simulink model "adm"  (R2020a)
settings: Solver=FixedStepAuto  StartTime=0.0  StopTime=2  FixedStep=0.00005  RelTol=1e-3
libraries: simulink x14, fuzblock x3
settings Model: Creator=13228  LastModifiedBy=13228
settings SolverCC: ZeroCrossAlgorithm=Adaptive

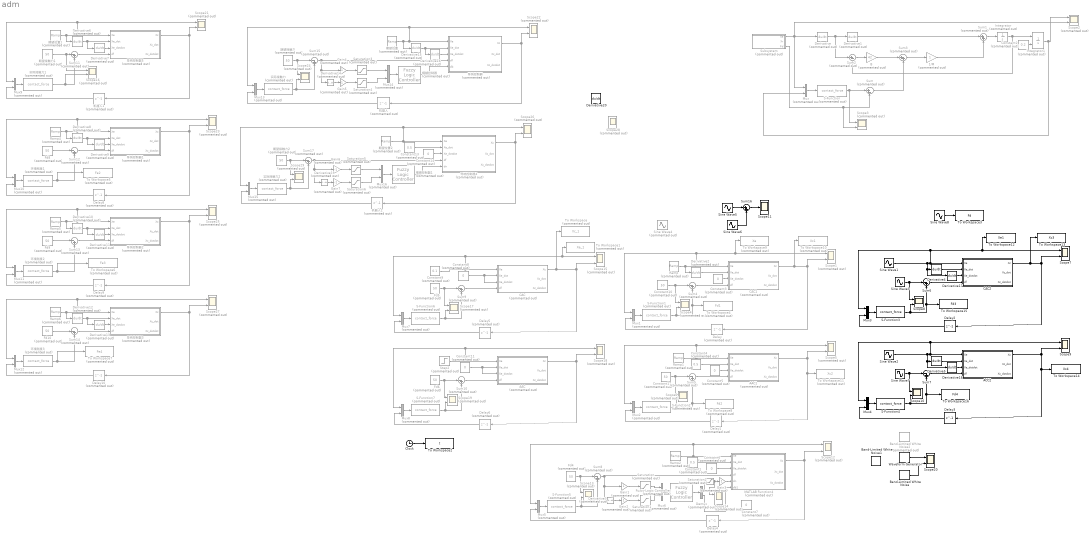
== system adm ==
  1/M : Gain  Commented=on
  AAC : MATLAB Function  Commented=on  TreatAsAtomicUnit=on
  AAC1 : MATLAB Function  Commented=on  TreatAsAtomicUnit=on
  ACC2 : MATLAB Function  TreatAsAtomicUnit=on
  B : Gain  Commented=on  Gain=42
  Band-Limited White Noise : simulink/Sources/Band-Limited White Noise  Cov=[0.2*0.2*0.01]  Ts=0.01  seed=[23341]
  Band-Limited White Noise1 : simulink/Sources/Band-Limited White Noise  Cov=[0.1]  Ts=0.1  seed=[23341]
  Band-Limited White Noise2 : simulink/Sources/Band-Limited White Noise  Commented=on  Cov=[0.1]  Ts=0.1  seed=[23341]
  CAC : MATLAB Function  Commented=on  TreatAsAtomicUnit=on
  CAC1 : MATLAB Function  Commented=on  TreatAsAtomicUnit=on
  CAC2 : MATLAB Function  TreatAsAtomicUnit=on
  Clock : Clock
  Constant1 : Constant  Commented=on  Value=0.5
  Constant10 : Constant  Commented=on  Value=50
  Constant{3,5..8,11,14} (7 alike) : Constant  Commented=on  Value=0
  Constant12 : Constant  Commented=on  Value=50
  Constant13 : Constant  Commented=on  Value=0.5
  Constant2 : Constant  Commented=on  Value=0.2
  Constant4 : Constant  Commented=on  Value=0.5
  Constant9 : Constant  Commented=on  Value=0.1
  Delay{,1,4,8..10} (6 alike) : Delay  Commented=on  DelayLength=1  InitialCondition=-0.002
  Delay2 : Delay  DelayLength=1  InitialCondition=0.098
  Delay3 : Delay  DelayLength=1  InitialCondition=0.098
  Delay5 : Delay  Commented=on  DelayLength=1  InitialCondition=0.098
  Delay6 : Delay  Commented=on  DelayLength=1  InitialCondition=0.098
  Demux : Demux  Commented=on  Outputs=2
  Derivative{,1..3,6..16,19} (16 alike) : Derivative  Commented=on
  Derivative{4..5,17..18,20} (5 alike) : Derivative
  Fd{4..6,8..10} (6 alike) : Constant  Commented=on  Value=50
  Fuzzy Logic Controller : fuzblock/Fuzzy Logic  Controller  Commented=on  FIS='fuzzy.fis'  OutputSampleNumber=101  DataType=double  FuzzifiedInputs=off  RuleFiringStrengths=off  RuleOutputs=off  AggregatedOutputs=off  SimulateUsing=Interpreted execution  OutOfRangeInputValueMessage=warning  NoRuleFiredMessage=warning  EmptyOutputFuzzySetMessage=warning
  Gain{1..5} (5 alike) : Gain  Commented=on
  Gain6 : Gain  Commented=on  Gain=-1
  Gain7 : Gain  Commented=on  Gain=-1
  Integrator : Integrator  Commented=on
  Integrator1 : Integrator  Commented=on  InitialConditionSource=external
  MATLAB Function4 : MATLAB Function  Commented=on  TreatAsAtomicUnit=on
  Mux{,1..2,5..16} (15 alike) : Mux  Commented=on  Inputs=2
  Mux3 : Mux  Inputs=2
  Mux4 : Mux  Inputs=2
  Ramp{,1..2,4..6} (6 alike) : simulink/Sources/Ramp  Commented=on  slope=0.5  start=0.001  InitialOutput=0
  S-Function{,1..2,5..7} (6 alike) : S-Function  Commented=on  FunctionName=contact_force  SFunctionDeploymentMode=off  EnableBusSupport=off
  S-Function3 : S-Function  FunctionName=contact_force  SFunctionDeploymentMode=off  EnableBusSupport=off
  S-Function4 : S-Function  FunctionName=contact_force  SFunctionDeploymentMode=off  EnableBusSupport=off
  Saturation{,1,3..4} (4 alike) : Saturate  Commented=on  UpperLimit=8  LowerLimit=-8
  Saturation2 : Saturate  Commented=on  UpperLimit=10000  LowerLimit=-10000
  Saturation5 : Saturate  Commented=on  UpperLimit=6  LowerLimit=-6
  Saturation6 : Saturate  Commented=on  UpperLimit=6  LowerLimit=-6
  Scope{1..6,12..19,21..27,29} (22 alike) : Scope  Commented=on  NumInputPorts=2
  Scope{7..10,20} (5 alike) : Scope  NumInputPorts=2
  Scope11 : Scope
  Scope28 : Scope  Commented=on
  Sine Wave1 : Sin  Amplitude=0.1  Bias=0.1  Frequency=pi  Phase=0.01  SampleTime=0
  Sine Wave2 : Sin  Amplitude=0.1  Bias=0.1  Frequency=pi  Phase=0.01  SampleTime=0
  Sine Wave3 : Sin  Amplitude=5  Bias=10  Frequency=pi  Phase=0.01  SampleTime=0
  Sine Wave4 : Sin  Commented=on  Amplitude=5  Bias=10  Frequency=2*pi  Phase=0.01  SampleTime=0
  Sine Wave5 : Sin  Amplitude=0.05  Bias=0.1  Frequency=2*pi  Phase=0.01  SampleTime=0
  Sine Wave6 : Sin  Amplitude=0.03  Bias=-0.1  Frequency=5*pi  Phase=pi  SampleTime=0
  Sine Wave7 : Sin  Amplitude=5  Bias=10  Frequency=pi  Phase=0.01  SampleTime=0
  Sine Wave8 : Sin  Amplitude=5  Bias=10  Frequency=pi  Phase=0.01  SampleTime=0
  Step2 : Step  Commented=on  Time=0  After=0.1  SampleTime=0
  Subsystem : Subsystem  Commented=on
  Sum : Sum  Commented=on  Inputs=|+-
  Sum1 : Sum  Commented=on  Inputs=|++
  Sum{4..5,8..15,17} (11 alike) : Sum  Commented=on  Inputs=|-+
  Sum16 : Sum  Inputs=|++
  Sum2 : Sum  Commented=on  Inputs=|+-
  Sum3 : Sum  Commented=on  Inputs=|++
  Sum6 : Sum  Inputs=|-+
  Sum7 : Sum  Inputs=|-+
  To Workspace : ToWorkspace  Commented=on  VariableName=Xc_1  SaveFormat=Timeseries  SampleTime=-1
  To Workspace1 : ToWorkspace  Commented=on  VariableName=Xe_1  SaveFormat=Timeseries  SampleTime=-1
  To Workspace10 : ToWorkspace  Commented=on  VariableName=Xc1  SaveFormat=Timeseries  SampleTime=-1
  To Workspace11 : ToWorkspace  Commented=on  VariableName=Xc2  SaveFormat=Timeseries  SampleTime=-1
  To Workspace12 : ToWorkspace  VariableName=Xe1  SaveFormat=Timeseries  SampleTime=-1
  To Workspace13 : ToWorkspace  VariableName=Xc3  SaveFormat=Timeseries  SampleTime=-1
  To Workspace14 : ToWorkspace  VariableName=Xc4  SaveFormat=Timeseries  SampleTime=-1
  To Workspace15 : ToWorkspace  VariableName=Fd3  SaveFormat=Timeseries  SampleTime=-1
  To Workspace16 : ToWorkspace  VariableName=Fd4  SaveFormat=Timeseries  SampleTime=-1
  To Workspace2 : ToWorkspace  VariableName=t  SaveFormat=Timeseries  SampleTime=-1
  To Workspace3 : ToWorkspace  VariableName=Fd  SaveFormat=Timeseries  SampleTime=-1
  To Workspace4 : ToWorkspace  Commented=on  VariableName=Fd1  SaveFormat=Timeseries  SampleTime=-1
  To Workspace5 : ToWorkspace  Commented=on  VariableName=Fe2  SaveFormat=Timeseries  SampleTime=-1
  To Workspace6 : ToWorkspace  Commented=on  VariableName=Fe3  SaveFormat=Timeseries  SampleTime=-1
  To Workspace7 : ToWorkspace  Commented=on  VariableName=Fe4  SaveFormat=Timeseries  SampleTime=-1
  To Workspace8 : ToWorkspace  Commented=on  VariableName=Fd2  SaveFormat=Timeseries  SampleTime=-1
  To Workspace9 : ToWorkspace  Commented=on  VariableName=Xe  SaveFormat=Timeseries  SampleTime=-1
  Waveform Generator : simulink/Sources/Waveform Generator  OutMin=[]  OutMax=[]  OutDataTypeStr=double  SelectedSignal=1  BlockNames=MultiportSwitch_e3df3653d217406  SampleTime=0.1
  实际接触力 : S-Function  Commented=on  FunctionName=contact_force  SFunctionDeploymentMode=off  EnableBusSupport=off
  实际接触力1 : S-Function  Commented=on  FunctionName=contact_force  SFunctionDeploymentMode=off  EnableBusSupport=off
  实际接触力2 : S-Function  Commented=on  FunctionName=contact_force  SFunctionDeploymentMode=off  EnableBusSupport=off
  导纳控制器 : MATLAB Function  Commented=on  TreatAsAtomicUnit=on
  导纳控制器1 : MATLAB Function  Commented=on  TreatAsAtomicUnit=on
  导纳控制器2 : MATLAB Function  Commented=on  TreatAsAtomicUnit=on
  导纳控制器3 : MATLAB Function  Commented=on  TreatAsAtomicUnit=on
  导纳控制器4 : MATLAB Function  Commented=on  TreatAsAtomicUnit=on
  导纳控制器5 : MATLAB Function  Commented=on  TreatAsAtomicUnit=on
  期望位置 : simulink/Sources/Ramp  Commented=on  slope=0.5  start=0.001  InitialOutput=0
  期望位置1 : simulink/Sources/Ramp  Commented=on  slope=0.5  start=0.001  InitialOutput=0
  期望位置2 : simulink/Sources/Ramp  Commented=on  slope=0.5  start=0.001  InitialOutput=0
  期望接触力 : Constant  Commented=on  Value=50
  期望接触力1 : Constant  Commented=on  Value=50
  期望接触力2 : Constant  Commented=on  Value=50
  机器人 : Delay  Commented=on  DelayLength=1  InitialCondition=-0.002
  机器人1 : Delay  Commented=on  DelayLength=1  InitialCondition=-0.002
  机器人2 : Delay  Commented=on  DelayLength=1  InitialCondition=-0.002
  模糊控制器 : fuzblock/Fuzzy Logic  Controller  Commented=on  FIS='fuzzy3.fis'  OutputSampleNumber=101  DataType=double  FuzzifiedInputs=off  RuleFiringStrengths=off  RuleOutputs=off  AggregatedOutputs=off  SimulateUsing=Interpreted execution  OutOfRangeInputValueMessage=warning  NoRuleFiredMessage=warning  EmptyOutputFuzzySetMessage=warning
  模糊控制器1 : fuzblock/Fuzzy Logic  Controller  Commented=on  FIS='fuzzy_a.fis'  OutputSampleNumber=101  DataType=double  FuzzifiedInputs=off  RuleFiringStrengths=off  RuleOutputs=off  AggregatedOutputs=off  SimulateUsing=Interpreted execution  OutOfRangeInputValueMessage=warning  NoRuleFiredMessage=warning  EmptyOutputFuzzySetMessage=warning
  环境刚度1 : S-Function  Commented=on  FunctionName=contact_force  SFunctionDeploymentMode=off  EnableBusSupport=off
  环境刚度2 : S-Function  Commented=on  FunctionName=contact_force  SFunctionDeploymentMode=off  EnableBusSupport=off
  环境刚度3 : S-Function  Commented=on  FunctionName=contact_force  SFunctionDeploymentMode=off  EnableBusSupport=off
  wires:
  S-Function/1 -> Scope3/1, Sum/1
  Mux/1 -> S-Function/1
  Subsystem/1(Xe) -> Scope2/2, Derivative/1, Mux/1
  CAC1/1(Xc) -> To Workspace10/1, Scope1/2, Delay/1
  Derivative/1 -> Sum2/1, Derivative1/1
  Derivative1/1 -> Sum1/1
  Sum1/1 -> Integrator/1
  Subsystem/3(Fd) -> Scope3/2, Sum/2
  Integrator/1 -> Integrator1/1, Sum2/2
  Sum2/1 -> B/1
  B/1 -> Sum3/1
  Sum/1 -> Sum3/2
  Sum3/1 -> 1/M/1
  1/M/1 -> Sum1/2
  Constant2/1 -> Integrator1/2
  Integrator1/1 -> Mux/2, Scope2/1
  Mux1/1 -> S-Function1/1
  Constant10/1 -> Scope4/1, Sum4/1
  S-Function1/1 -> Scope4/2, To Workspace4/1, Sum4/2
  Sum4/1 -> CAC1/4(df)
  Delay/1 -> Mux1/2
  Ramp/1 -> Derivative2/1, Mux1/1, To Workspace9/1, Scope1/1, CAC1/1(Xe)
  Derivative2/1 -> CAC1/2(Xe_dot)
  Ramp1/1 -> Mux2/1, Scope5/1, AAC1/1(Xe)
  Mux2/1 -> S-Function2/1
  S-Function2/1 -> Scope6/2, To Workspace8/1, Sum5/2
  Constant12/1 -> Scope6/1, Sum5/1
  Delay1/1 -> Mux2/2
  Sum5/1 -> AAC1/4(df)
  S-Function4/1 -> Scope10/2, To Workspace16/1, Sum7/2
  Sine Wave1/1 -> Mux3/1, To Workspace12/1, Scope7/1, CAC2/1(Xe), Derivative17/1, Derivative4/1
  ACC2/1(Xc) -> Scope9/2, To Workspace14/1, Delay3/1
  Mux3/1 -> S-Function3/1
  Derivative5/1 -> ACC2/2(Xe_dot)
  Sum7/1 -> ACC2/4(df)
  Mux4/1 -> S-Function4/1
  Delay3/1 -> Mux4/2
  Delay2/1 -> Mux3/2
  Sine Wave7/1 -> Scope10/1, Sum7/1
  Derivative4/1 -> CAC2/2(Xe_dot)
  Sine Wave2/1 -> ACC2/1(Xe), Mux4/1, Scope9/1, Derivative18/1, Derivative5/1
  Sum6/1 -> CAC2/4(df)
  S-Function3/1 -> Scope8/2, To Workspace15/1, Sum6/2
  Sine Wave3/1 -> Scope8/1, Sum6/1
  CAC2/1(Xc) -> To Workspace13/1, Scope7/2, Delay2/1
  Constant3/1 -> CAC1/3(Xe_dotdot)
  Constant4/1 -> AAC1/2(Xe_dot)
  Constant5/1 -> AAC1/3(Xe_dotdot)
  Constant1/1 -> MATLAB Function4/2(Xe_dot)
  Constant6/1 -> MATLAB Function4/3(Xe_dotdot)
  MATLAB Function4/1(Xc) -> Scope12/2, Delay4/1
  Mux5/1 -> S-Function5/1
  Delay4/1 -> Mux5/2
  Fd4/1 -> Scope13/1, Sum8/1
  S-Function5/1 -> Scope13/2, Sum8/2
  Sum8/1 -> Gain1/1, Derivative3/1, MATLAB Function4/4(df)
  Ramp2/1 -> Mux5/1, Scope12/1, MATLAB Function4/1(Xe)
  Gain1/1 -> Saturation/1
  Gain2/1 -> Saturation1/1
  Derivative3/1 -> Gain2/1
  Saturation/1 -> Mux6/1
  Saturation1/1 -> Mux6/2
  Mux6/1 -> Fuzzy Logic Controller/1
  Fuzzy Logic Controller/1 -> Demux/1
  Demux/2 -> MATLAB Function4/6(db1)
  Demux/1 -> Saturation2/1
  Gain3/1 -> MATLAB Function4/5(dn)
  Saturation2/1 -> Scope14/1, Gain3/1
  Sum10/1 -> AAC/4(df)
  Step2/1 -> Mux8/1, Scope18/1, AAC/1(Xe)
  Mux7/1 -> S-Function6/1
  Fd6/1 -> Scope19/1, Sum10/1
  S-Function7/1 -> Scope19/2, Sum10/2
  Constant11/1 -> AAC/3(Xe_dotdot), AAC/2(Xe_dot)
  S-Function6/1 -> Scope17/2, Sum9/2
  Constant9/1 -> Mux7/1, To Workspace1/1, Scope15/1, CAC/1(Xe)
  Fd5/1 -> Scope17/1, Sum9/1
  Sum9/1 -> CAC/4(df)
  Mux8/1 -> S-Function7/1
  CAC/1(Xc) -> To Workspace/1, Scope15/2, Delay5/1
  Delay6/1 -> Mux8/2
  Delay5/1 -> Mux7/2
  Constant8/1 -> CAC/3(Xe_dotdot), CAC/2(Xe_dot)
  AAC/1(Xc) -> Scope18/2, Delay6/1
  Clock/1 -> To Workspace2/1
  Waveform Generator/1 -> Scope20/1
  Band-Limited White Noise/1 -> Scope20/2
  Derivative7/1 -> 导纳控制器5/3(Xe_dotdot)
  实际接触力1/1 -> Scope16/2, Sum11/2
  机器人1/1 -> Mux9/2
  Sum11/1 -> 导纳控制器5/4(df)
  期望位置1/1 -> Derivative6/1, Mux9/1, Scope21/1, 导纳控制器5/1(Xe)
  Mux9/1 -> 实际接触力1/1
  导纳控制器5/1(Xc) -> Scope21/2, 机器人1/1
  Derivative6/1 -> Derivative7/1, 导纳控制器5/2(Xe_dot)
  期望接触力1/1 -> Scope16/1, Sum11/1
  Derivative8/1 -> Derivative9/1, 导纳控制器1/2(Xe_dot)
  Mux10/1 -> 环境刚度1/1
  Ramp4/1 -> Derivative8/1, Mux10/1, Scope23/1, 导纳控制器1/1(Xe)
  导纳控制器1/1(Xc) -> Scope23/2, Delay8/1
  Delay8/1 -> Mux10/2
  Fd8/1 -> Sum12/1
  环境刚度1/1 -> To Workspace5/1, Sum12/2
  Derivative9/1 -> 导纳控制器1/3(Xe_dotdot)
  Sum12/1 -> 导纳控制器1/4(df)
  Derivative10/1 -> Derivative11/1, 导纳控制器2/2(Xe_dot)
  Mux11/1 -> 环境刚度2/1
  Ramp5/1 -> Derivative10/1, Mux11/1, Scope25/1, 导纳控制器2/1(Xe)
  导纳控制器2/1(Xc) -> Scope25/2, Delay9/1
  Delay9/1 -> Mux11/2
  Fd9/1 -> Sum13/1
  环境刚度2/1 -> To Workspace6/1, Sum13/2
  Derivative11/1 -> 导纳控制器2/3(Xe_dotdot)
  Sum13/1 -> 导纳控制器2/4(df)
  Derivative12/1 -> Derivative13/1, 导纳控制器3/2(Xe_dot)
  Mux12/1 -> 环境刚度3/1
  Ramp6/1 -> Derivative12/1, Mux12/1, Scope27/1, 导纳控制器3/1(Xe)
  导纳控制器3/1(Xc) -> Scope27/2, Delay10/1
  Delay10/1 -> Mux12/2
  Fd10/1 -> Sum14/1
  环境刚度3/1 -> To Workspace7/1, Sum14/2
  Derivative13/1 -> 导纳控制器3/3(Xe_dotdot)
  Sum14/1 -> 导纳控制器3/4(df)
  实际接触力/1 -> Sum15/2, Scope24/2
  期望位置/1 -> Derivative15/1, Mux13/1, Scope22/1, 导纳控制器/1(Xe)
  Mux14/1 -> 模糊控制器/1
  Gain5/1 -> Saturation4/1
  Gain4/1 -> Saturation3/1
  Sum15/1 -> Gain4/1, Derivative14/1, 导纳控制器/4(df)
  期望接触力/1 -> Scope24/1, Sum15/1
  导纳控制器/1(Xc) -> Scope22/2, 机器人/1
  Derivative14/1 -> Gain5/1
  Mux13/1 -> 实际接触力/1
  机器人/1 -> Mux13/2
  Saturation3/1 -> Mux14/1
  Saturation4/1 -> Mux14/2
  模糊控制器/1 -> 导纳控制器/5(db)
  Derivative15/1 -> Derivative16/1, 导纳控制器/2(Xe_dot)
  Derivative16/1 -> 导纳控制器/3(Xe_dotdot)
  AAC1/1(Xc) -> Scope5/2, To Workspace11/1, Delay1/1
  Sine Wave5/1 -> Sum16/1
  Sum16/1 -> Scope11/1
  Sine Wave6/1 -> Sum16/2
  Derivative17/1 -> CAC2/3(Xe_dotdot)
  Derivative18/1 -> ACC2/3(Xe_dotdot)
  Sine Wave8/1 -> To Workspace3/1
  模糊控制器1/1 -> 导纳控制器4/5(dn)
  Saturation5/1 -> Mux16/1
  导纳控制器4/1(Xc) -> Scope26/2, 机器人2/1
  Constant13/1 -> 导纳控制器4/2(Xe_dot)
  Saturation6/1 -> Mux16/2
  机器人2/1 -> Mux15/2
  期望接触力2/1 -> Scope29/1, Sum17/1
  Derivative19/1 -> Gain7/1
  期望位置2/1 -> Mux15/1, Scope26/1, 导纳控制器4/1(Xe)
  Mux15/1 -> 实际接触力2/1
  Sum17/1 -> Gain6/1, Derivative19/1, 导纳控制器4/4(df)
  实际接触力2/1 -> Sum17/2, Scope29/2
  Constant14/1 -> 导纳控制器4/3(Xe_dotdot)
  Gain6/1 -> Saturation5/1
  Mux16/1 -> 模糊控制器1/1
  Gain7/1 -> Saturation6/1

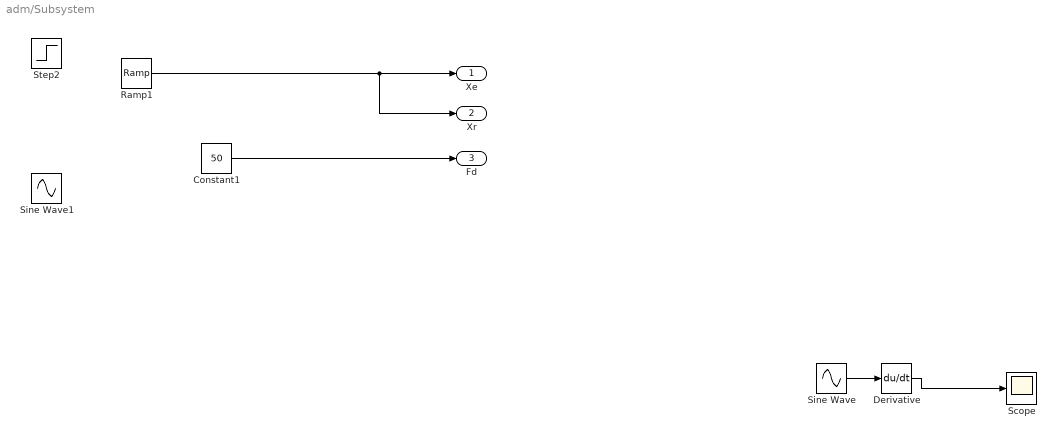
== system adm/Subsystem ==
  Constant1 : Constant  Value=50
  Derivative : Derivative
  Ramp1 : simulink/Sources/Ramp  slope=0.5  start=0.01  InitialOutput=0
  Scope : Scope
  Sine Wave : Sin  SampleTime=0
  Sine Wave1 : Sin  Bias=-1  Phase=pi / 2  SampleTime=0
  Step2 : Step  Time=0  After=0.1  SampleTime=0
  Xe : Outport
  Xr : Outport  Port=2
  Fd : Outport  Port=3
  wires:
  Constant1/1 -> Fd/1
  Ramp1/1 -> Xr/1, Xe/1
  Sine Wave/1 -> Derivative/1
  Derivative/1 -> Scope/1

== matlab function adm/导纳控制器5 ==
  settings: updateMethod=DISCRETE
  data: Xe input; Xc output; Xe_dot input; Xe_dotdot input; df input; Xc_dot output; Xc_dotdot output
function [Xc,Xc_dot,Xc_dotdot]  = fcnlmp(Xe,Xe_dot,Xe_dotdot,df)  
	m =1;b = 50;k=10;T = 0.00005; % 参数初始化  
	persistent Xc_pre Xc_dot_pre;% 持久变量 https://ww2.mathworks.cn/help/matlab/ref/persistent.html  
	if isempty(Xc_pre)   
	   Xc_pre = -0.002;  
	end  
	if isempty(Xc_dot_pre)   
	   Xc_dot_pre = 0;  
	end  
	Xc_dotdot_pre = Xe_dotdot + 1/m*(df + b*(Xe_dot - Xc_dot_pre) + k*(Xe - Xc_pre)); % 上一采样时间 nT 机器人末端的实际运动加速度  
	Xc = Xc_pre + Xc_dot_pre*T;           % 当前采样时间 (n+1)T 机器人末端的实际运动位置  
	Xc_dot = Xc_dot_pre + Xc_dotdot_pre*T;% 当前采样时间 (n+1)T 机器人末端的实际运动速度  
	Xc_dotdot = Xc_dotdot_pre;            % 当前采样时间 (n+1)T 机器人末端的实际运动加速度  
	Xc_dot_pre = Xc_dot;                  % 上一采样时间 nT 机器人末端的实际运动速度  
	Xc_pre = Xc;                          % 上一采样时间 nT 机器人末端的实际运动位置  
end

== matlab function adm/导纳控制器1 ==
  settings: updateMethod=DISCRETE
  data: Xe input; Xc output; Xe_dot input; Xe_dotdot input; df input; Xc_dot output; Xc_dotdot output
function [Xc,Xc_dot,Xc_dotdot]  = fcnlmp(Xe,Xe_dot,Xe_dotdot,df)  
	m =1;b = 50;k=10;T = 0.00005; % 参数初始化  
	persistent Xc_pre Xc_dot_pre;% 持久变量 https://ww2.mathworks.cn/help/matlab/ref/persistent.html  
	if isempty(Xc_pre)   
	   Xc_pre = -0.002;  
	end  
	if isempty(Xc_dot_pre)   
	   Xc_dot_pre = 0;  
	end  
	Xc_dotdot_pre = Xe_dotdot + 1/m*(df + b*(Xe_dot - Xc_dot_pre) + k*(Xe - Xc_pre)); % 上一采样时间 nT 机器人末端的实际运动加速度  
	Xc = Xc_pre + Xc_dot_pre*T;           % 当前采样时间 (n+1)T 机器人末端的实际运动位置  
	Xc_dot = Xc_dot_pre + Xc_dotdot_pre*T;% 当前采样时间 (n+1)T 机器人末端的实际运动速度  
	Xc_dotdot = Xc_dotdot_pre;            % 当前采样时间 (n+1)T 机器人末端的实际运动加速度  
	Xc_dot_pre = Xc_dot;                  % 上一采样时间 nT 机器人末端的实际运动速度  
	Xc_pre = Xc;                          % 上一采样时间 nT 机器人末端的实际运动位置  
end

== matlab function adm/导纳控制器2 ==
  settings: updateMethod=DISCRETE
  data: Xe input; Xc output; Xe_dot input; Xe_dotdot input; df input; Xc_dot output; Xc_dotdot output
function [Xc,Xc_dot,Xc_dotdot]  = fcnlmp(Xe,Xe_dot,Xe_dotdot,df)  
	m =1;b = 130;k=10;T = 0.00005; % 参数初始化  
	persistent Xc_pre Xc_dot_pre;% 持久变量 https://ww2.mathworks.cn/help/matlab/ref/persistent.html  
	if isempty(Xc_pre)   
	   Xc_pre = -0.002;  
	end  
	if isempty(Xc_dot_pre)   
	   Xc_dot_pre = 0;  
	end  
	Xc_dotdot_pre = Xe_dotdot + 1/m*(df + b*(Xe_dot - Xc_dot_pre) + k*(Xe - Xc_pre)); % 上一采样时间 nT 机器人末端的实际运动加速度  
	Xc = Xc_pre + Xc_dot_pre*T;           % 当前采样时间 (n+1)T 机器人末端的实际运动位置  
	Xc_dot = Xc_dot_pre + Xc_dotdot_pre*T;% 当前采样时间 (n+1)T 机器人末端的实际运动速度  
	Xc_dotdot = Xc_dotdot_pre;            % 当前采样时间 (n+1)T 机器人末端的实际运动加速度  
	Xc_dot_pre = Xc_dot;                  % 上一采样时间 nT 机器人末端的实际运动速度  
	Xc_pre = Xc;                          % 上一采样时间 nT 机器人末端的实际运动位置  
end

== matlab function adm/导纳控制器3 ==
  settings: updateMethod=DISCRETE
  data: Xe input; Xc output; Xe_dot input; Xe_dotdot input; df input; Xc_dot output; Xc_dotdot output
function [Xc,Xc_dot,Xc_dotdot]  = fcnlmp(Xe,Xe_dot,Xe_dotdot,df)  
	m =1;b = 60;k=500;T = 0.00005; % 参数初始化  
	persistent Xc_pre Xc_dot_pre;% 持久变量 https://ww2.mathworks.cn/help/matlab/ref/persistent.html  
	if isempty(Xc_pre)   
	   Xc_pre = -0.002;  
	end  
	if isempty(Xc_dot_pre)   
	   Xc_dot_pre = 0;  
	end  
	Xc_dotdot_pre = Xe_dotdot + 1/m*(df + b*(Xe_dot - Xc_dot_pre) + k*(Xe - Xc_pre)); % 上一采样时间 nT 机器人末端的实际运动加速度  
	Xc = Xc_pre + Xc_dot_pre*T;           % 当前采样时间 (n+1)T 机器人末端的实际运动位置  
	Xc_dot = Xc_dot_pre + Xc_dotdot_pre*T;% 当前采样时间 (n+1)T 机器人末端的实际运动速度  
	Xc_dotdot = Xc_dotdot_pre;            % 当前采样时间 (n+1)T 机器人末端的实际运动加速度  
	Xc_dot_pre = Xc_dot;                  % 上一采样时间 nT 机器人末端的实际运动速度  
	Xc_pre = Xc;                          % 上一采样时间 nT 机器人末端的实际运动位置  
end

== matlab function adm/导纳控制器 ==
  settings: updateMethod=DISCRETE
  data: Xe input; Xc output; Xe_dot input; Xe_dotdot input; df input; Xc_dot output; Xc_dotdot output; db input
function [Xc,Xc_dot,Xc_dotdot]  = fcnlmp(Xe,Xe_dot,Xe_dotdot,df,db)  
	m =1;b = 60;k=0;T = 0.00005;a=0.01; % 参数初始化  
	persistent Xc_pre Xc_dot_pre ;% 持久变量 https://ww2.mathworks.cn/help/matlab/ref/persistent.html  
	if isempty(Xc_pre)   
	   Xc_pre = -0.002;  
	end  
	if isempty(Xc_dot_pre)   
	   Xc_dot_pre = 0;  
    end  
% 	E=-(Xe_dot - Xc_dot_pre);
    Xc_dotdot_pre = Xe_dotdot + 1/m*(df + (b + db)*(Xe_dot - Xc_dot_pre) + k*(Xe - Xc_pre)); % 上一采样时间 nT 机器人末端的实际运动加速度  
% 	Xc_dotdot_pre = Xe_dotdot + 1/m*df;
    Xc = Xc_pre + Xc_dot_pre*T;           % 当前采样时间 (n+1)T 机器人末端的实际运动位置  
	Xc_dot = Xc_dot_pre + Xc_dotdot_pre*T;% 当前采样时间 (n+1)T 机器人末端的实际运动速度  
	Xc_dotdot = Xc_dotdot_pre;            % 当前采样时间 (n+1)T 机器人末端的实际运动加速度  
	Xc_dot_pre = Xc_dot;                  % 上一采样时间 nT 机器人末端的实际运动速度  
	Xc_pre = Xc;                          % 上一采样时间 nT 机器人末端的实际运动位置  
    B=b+db;
    
end

== matlab function adm/导纳控制器4 ==
  settings: updateMethod=DISCRETE
  data: Xe input; Xc output; Xe_dot input; Xe_dotdot input; df input; Xc_dot output; Xc_dotdot output; dn input
function [Xc,Xc_dot,Xc_dotdot]  = fcnlmp(Xe,Xe_dot,Xe_dotdot,df,dn)  
	m =1;b = 65;k=0;T = 0.0005;a=0.01; % 参数初始化  
	persistent Xc_pre Xc_dot_pre df_pre fi_pre;% 持久变量 https://ww2.mathworks.cn/help/matlab/ref/persistent.html  
	if isempty(Xc_pre)   
	   Xc_pre = -0.002;  
	end  
	if isempty(Xc_dot_pre)   
	   Xc_dot_pre = 0.1;  
    end  
    if isempty(df_pre)   
	   df_pre = 51;  
    end  
    if isempty(fi_pre)   
	   fi_pre = 0;  
    end  
    fi = fi_pre + (a + dn) /b * df_pre;
%     fi = fi_pre + (a) /b * df_pre;
    db = fi * b/(Xe_dot - Xc_dot_pre);
    fprintf('fi=%f,db=%f\n',fi,db);
    fi_pre = fi;
    df_pre = df;
%     db = 0;   
	Xc_dotdot_pre = Xe_dotdot + 1/m*(df + (b + db)*(Xe_dot - Xc_dot_pre) + k*(Xe - Xc_pre)); % 上一采样时间 nT 机器人末端的实际运动加速度  
	Xc = Xc_pre + Xc_dot_pre*T;           % 当前采样时间 (n+1)T 机器人末端的实际运动位置  
	Xc_dot = Xc_dot_pre + Xc_dotdot_pre*T;% 当前采样时间 (n+1)T 机器人末端的实际运动速度  
	Xc_dotdot = Xc_dotdot_pre;            % 当前采样时间 (n+1)T 机器人末端的实际运动加速度  
	Xc_dot_pre = Xc_dot;                  % 上一采样时间 nT 机器人末端的实际运动速度  
	Xc_pre = Xc;                          % 上一采样时间 nT 机器人末端的实际运动位置  
end

== matlab function adm/AAC1 ==
  settings: updateMethod=DISCRETE
  data: Xe input; Xc output; Xe_dot input; Xe_dotdot input; df input; Xc_dot output; Xc_dotdot output
function [Xc,Xc_dot,Xc_dotdot]  = fcnlmp(Xe,Xe_dot,Xe_dotdot,df)  
	m =1;b = 60;k=0;T = 0.0005;a=0.01; % 参数初始化  
	persistent Xc_pre Xc_dot_pre df_pre fi_pre;% 持久变量 https://ww2.mathworks.cn/help/matlab/ref/persistent.html  
	if isempty(Xc_pre)   
	   Xc_pre = -0.002;  
	end  
	if isempty(Xc_dot_pre)   
	   Xc_dot_pre = 0.1;  
    end  
    if isempty(df_pre)   
	   df_pre = 51;  
    end  
    if isempty(fi_pre)   
	   fi_pre = 0;  
    end  
    fi = fi_pre + a/b * df_pre;
    db = fi * b/(Xe_dot - Xc_dot_pre);
    fprintf('fi=%f,db=%f\n',fi,db);
    fi_pre = fi;
    df_pre = df;
%     db = 0;   
	Xc_dotdot_pre = Xe_dotdot + 1/m*(df + (b + db)*(Xe_dot - Xc_dot_pre) + k*(Xe - Xc_pre)); % 上一采样时间 nT 机器人末端的实际运动加速度  
	Xc = Xc_pre + Xc_dot_pre*T;           % 当前采样时间 (n+1)T 机器人末端的实际运动位置  
	Xc_dot = Xc_dot_pre + Xc_dotdot_pre*T;% 当前采样时间 (n+1)T 机器人末端的实际运动速度  
	Xc_dotdot = Xc_dotdot_pre;            % 当前采样时间 (n+1)T 机器人末端的实际运动加速度  
	Xc_dot_pre = Xc_dot;                  % 上一采样时间 nT 机器人末端的实际运动速度  
	Xc_pre = Xc;                          % 上一采样时间 nT 机器人末端的实际运动位置  
end

== matlab function adm/CAC1 ==
  settings: updateMethod=DISCRETE
  data: Xe input; Xc output; Xe_dot input; Xe_dotdot input; df input; Xc_dot output; Xc_dotdot output
function [Xc,Xc_dot,Xc_dotdot]  = fcnlmp(Xe,Xe_dot,Xe_dotdot,df)  
	m =1;b = 60;k=0;T = 0.00005; % 参数初始化  
	persistent Xc_pre Xc_dot_pre;% 持久变量 https://ww2.mathworks.cn/help/matlab/ref/persistent.html  
	if isempty(Xc_pre)   
	   Xc_pre = -0.002;  
	end  
	if isempty(Xc_dot_pre)   
	   Xc_dot_pre = 0;  
	end  
	Xc_dotdot_pre = Xe_dotdot + 1/m*(df + b*(Xe_dot - Xc_dot_pre) + k*(Xe - Xc_pre)); % 上一采样时间 nT 机器人末端的实际运动加速度  
	Xc = Xc_pre + Xc_dot_pre*T;           % 当前采样时间 (n+1)T 机器人末端的实际运动位置  
	Xc_dot = Xc_dot_pre + Xc_dotdot_pre*T;% 当前采样时间 (n+1)T 机器人末端的实际运动速度  
	Xc_dotdot = Xc_dotdot_pre;            % 当前采样时间 (n+1)T 机器人末端的实际运动加速度  
	Xc_dot_pre = Xc_dot;                  % 上一采样时间 nT 机器人末端的实际运动速度  
	Xc_pre = Xc;                          % 上一采样时间 nT 机器人末端的实际运动位置  
end

== matlab function adm/CAC2 ==
  settings: updateMethod=DISCRETE
  data: Xe input; Xc output; Xe_dot input; Xe_dotdot input; df input; Xc_dot output; Xc_dotdot output
function [Xc,Xc_dot,Xc_dotdot]  = fcnlmp(Xe,Xe_dot,Xe_dotdot,df)  
	m =1;b = 60;k=0;T = 0.00005; % 参数初始化  
	persistent Xc_pre Xc_dot_pre;% 持久变量 https://ww2.mathworks.cn/help/matlab/ref/persistent.html  
	if isempty(Xc_pre)   
	   Xc_pre = 0.098;  
	end  
	if isempty(Xc_dot_pre)   
	   Xc_dot_pre = 0;  
	end  
	Xc_dotdot_pre = Xe_dotdot + 1/m*(df + b*(Xe_dot - Xc_dot_pre) + k*(Xe - Xc_pre)); % 上一采样时间 nT 机器人末端的实际运动加速度  
	Xc = Xc_pre + Xc_dot_pre*T;           % 当前采样时间 (n+1)T 机器人末端的实际运动位置  
	Xc_dot = Xc_dot_pre + Xc_dotdot_pre*T;% 当前采样时间 (n+1)T 机器人末端的实际运动速度  
	Xc_dotdot = Xc_dotdot_pre;            % 当前采样时间 (n+1)T 机器人末端的实际运动加速度  
	Xc_dot_pre = Xc_dot;                  % 上一采样时间 nT 机器人末端的实际运动速度  
	Xc_pre = Xc;                          % 上一采样时间 nT 机器人末端的实际运动位置  
end

== matlab function adm/ACC2 ==
  settings: updateMethod=DISCRETE
  data: Xe input; Xc output; Xe_dot input; Xe_dotdot input; df input; Xc_dot output; Xc_dotdot output
function [Xc,Xc_dot,Xc_dotdot]  = fcnlmp(Xe,Xe_dot,Xe_dotdot,df)  
	m =1;b = 60;k=0;T = 0.0005;a=0.01; % 参数初始化  
	persistent Xc_pre Xc_dot_pre df_pre fi_pre;% 持久变量 https://ww2.mathworks.cn/help/matlab/ref/persistent.html  
	if isempty(Xc_pre)   
	   Xc_pre = 0.098;  
	end  
	if isempty(Xc_dot_pre)   
	   Xc_dot_pre = 0.1;  
    end  
    if isempty(df_pre)   
	   df_pre = 51;  
    end  
    if isempty(fi_pre)   
	   fi_pre = 0;  
    end  
    fi = fi_pre + a/b * df_pre;
%     if (fi <= 0.01) && (fi >= -0.01) 
%         fi =  fi/abs(fi)* 0.01;
%     elseif (fi <= -1000) || (fi >= 1000) 
%         fi =  fi/abs(fi)* 1000;
%     end
    db = fi * b/(Xe_dot - Xc_dot_pre);
%     if (db <= 0.01) && (db >= -0.01) 
%         db =  db/abs(db)* 0.01;
%     elseif (db <= -1000) || (db >= 1000) 
%         db =  db/abs(db)* 1000;
%     end
    fprintf('fi=%f,db=%f\n',fi,db);
    fi_pre = fi;
    df_pre = df;
%     db = 0;   
	Xc_dotdot_pre = Xe_dotdot + 1/m*(df + (b + db)*(Xe_dot - Xc_dot_pre) + k*(Xe - Xc_pre)); % 上一采样时间 nT 机器人末端的实际运动加速度  
	Xc = Xc_pre + Xc_dot_pre*T;           % 当前采样时间 (n+1)T 机器人末端的实际运动位置  
	Xc_dot = Xc_dot_pre + Xc_dotdot_pre*T;% 当前采样时间 (n+1)T 机器人末端的实际运动速度  
	Xc_dotdot = Xc_dotdot_pre;            % 当前采样时间 (n+1)T 机器人末端的实际运动加速度  
	Xc_dot_pre = Xc_dot;                  % 上一采样时间 nT 机器人末端的实际运动速度  
	Xc_pre = Xc;                          % 上一采样时间 nT 机器人末端的实际运动位置  
end

== matlab function adm/MATLAB Function4 ==
  settings: updateMethod=DISCRETE
  data: Xe input; Xc output; Xe_dot input; Xe_dotdot input; df input; Xc_dot output; Xc_dotdot output; dn input; db1 input
function [Xc,Xc_dot,Xc_dotdot]  = fcnlmp(Xe,Xe_dot,Xe_dotdot,df,dn,db1)  
	m =1;b = 65;k=0;T = 0.005;a=0.01; % 参数初始化  
	persistent Xc_pre Xc_dot_pre df_pre fi_pre;% 持久变量 https://ww2.mathworks.cn/help/matlab/ref/persistent.html  
	if isempty(Xc_pre)   
	   Xc_pre = -0.002;  
	end  
	if isempty(Xc_dot_pre)   
	   Xc_dot_pre = 0.1;  
    end  
    if isempty(df_pre)   
	   df_pre = 51;  
    end  
    if isempty(fi_pre)   
	   fi_pre = 0;  
    end  
%     fi = fi_pre + (a+dn)/b * df_pre;
    fi = fi_pre + a/b * df_pre;
    db = fi * b/(Xe_dot - Xc_dot_pre);
    fprintf('fi=%f,db=%f\n',fi,db);
    fi_pre = fi;
    df_pre = df;
%     db = 0;   
	Xc_dotdot_pre = Xe_dotdot + 1/m*(df + (b + db+db1)*(Xe_dot - Xc_dot_pre) + k*(Xe - Xc_pre)); % 上一采样时间 nT 机器人末端的实际运动加速度  
	Xc = Xc_pre + Xc_dot_pre*T;           % 当前采样时间 (n+1)T 机器人末端的实际运动位置  
	Xc_dot = Xc_dot_pre + Xc_dotdot_pre*T;% 当前采样时间 (n+1)T 机器人末端的实际运动速度  
	Xc_dotdot = Xc_dotdot_pre;            % 当前采样时间 (n+1)T 机器人末端的实际运动加速度  
	Xc_dot_pre = Xc_dot;                  % 上一采样时间 nT 机器人末端的实际运动速度  
	Xc_pre = Xc;                          % 上一采样时间 nT 机器人末端的实际运动位置  
end

== matlab function adm/CAC ==
  settings: updateMethod=DISCRETE
  data: Xe input; Xc output; Xe_dot input; Xe_dotdot input; df input; Xc_dot output; Xc_dotdot output
function [Xc,Xc_dot,Xc_dotdot]  = fcnlmp(Xe,Xe_dot,Xe_dotdot,df)  
	m =1;b = 100;k=0;T = 0.00005; % 参数初始化  
	persistent Xc_pre Xc_dot_pre;% 持久变量 https://ww2.mathworks.cn/help/matlab/ref/persistent.html  
	if isempty(Xc_pre)   
	   Xc_pre = 0.098;  
	end  
	if isempty(Xc_dot_pre)   
	   Xc_dot_pre = 0;  
	end  
	Xc_dotdot_pre = Xe_dotdot + 1/m*(df + b*(Xe_dot - Xc_dot_pre) + k*(Xe - Xc_pre)); % 上一采样时间 nT 机器人末端的实际运动加速度  
	Xc = Xc_pre + Xc_dot_pre*T;           % 当前采样时间 (n+1)T 机器人末端的实际运动位置  
	Xc_dot = Xc_dot_pre + Xc_dotdot_pre*T;% 当前采样时间 (n+1)T 机器人末端的实际运动速度  
	Xc_dotdot = Xc_dotdot_pre;            % 当前采样时间 (n+1)T 机器人末端的实际运动加速度  
	Xc_dot_pre = Xc_dot;                  % 上一采样时间 nT 机器人末端的实际运动速度  
	Xc_pre = Xc;                          % 上一采样时间 nT 机器人末端的实际运动位置  
end

== matlab function adm/AAC ==
  settings: updateMethod=DISCRETE
  data: Xe input; Xc output; Xe_dot input; Xe_dotdot input; df input; Xc_dot output; Xc_dotdot output
function [Xc,Xc_dot,Xc_dotdot]  = fcnlmp(Xe,Xe_dot,Xe_dotdot,df)  
	m =1;b = 65;k=1000;T = 0.005;a=0.01; % 参数初始化  
	persistent Xc_pre Xc_dot_pre df_pre fi_pre;% 持久变量 https://ww2.mathworks.cn/help/matlab/ref/persistent.html  
	if isempty(Xc_pre)   
	   Xc_pre = 0.098;  
	end  
	if isempty(Xc_dot_pre)   
	   Xc_dot_pre = 0.1;  
    end  
    if isempty(df_pre)   
	   df_pre = 51;  
    end  
    if isempty(fi_pre)   
	   fi_pre = 0;  
    end  
    fi = fi_pre + a/b * df_pre;
    db = fi * b/(Xe_dot - Xc_dot_pre);
    fprintf('fi=%f,db=%f\n',fi,db);
    fi_pre = fi;
    df_pre = df;
%     db = 0;   
	Xc_dotdot_pre = Xe_dotdot + 1/m*(df + (b + db)*(Xe_dot - Xc_dot_pre) + k*(Xe - Xc_pre)); % 上一采样时间 nT 机器人末端的实际运动加速度  
	Xc = Xc_pre + Xc_dot_pre*T;           % 当前采样时间 (n+1)T 机器人末端的实际运动位置  
	Xc_dot = Xc_dot_pre + Xc_dotdot_pre*T;% 当前采样时间 (n+1)T 机器人末端的实际运动速度  
	Xc_dotdot = Xc_dotdot_pre;            % 当前采样时间 (n+1)T 机器人末端的实际运动加速度  
	Xc_dot_pre = Xc_dot;                  % 上一采样时间 nT 机器人末端的实际运动速度  
	Xc_pre = Xc;                          % 上一采样时间 nT 机器人末端的实际运动位置  
end
